simulink model "ElectricalSystems"  (R2020a)
settings: Solver=ode23t  StartTime=0.0  StopTime=10  RelTol=1e-3
undefined symbols (not defined in the file or in its folder): a, J, Ke, kt, kv, R, sigbuilder_block, Ts_motor, w0
libraries: fl_lib x54, nesl_utility x44, ee_lib x20, powerlib_meascontrol x16, fl_ps_legacy_lib x4, simulink x3
(part 2 of 2)

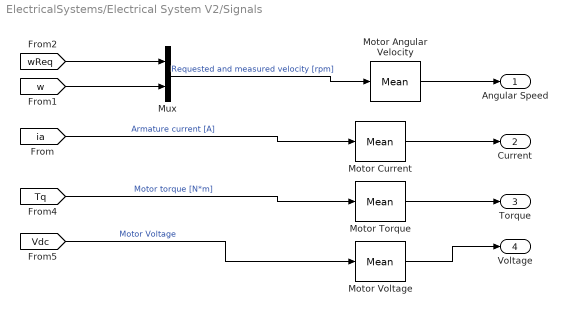
== system ElectricalSystems/Electrical System V2/Signals ==
  Motor Angular Velocity : powerlib_meascontrol/Measurements/Mean  Freq=100  Vinit=0  Ts=0
  Motor Current : powerlib_meascontrol/Measurements/Mean  Freq=100  Vinit=0  Ts=0
  Motor Torque : powerlib_meascontrol/Measurements/Mean  Freq=100  Vinit=0  Ts=0
  Motor Voltage : powerlib_meascontrol/Measurements/Mean  Freq=100  Vinit=0  Ts=0
  Mux : Mux  Inputs=2
  Angular Speed : Outport  VectorParamsAs1DForOutWhenUnconnected=off
  Current : Outport  Port=2  VectorParamsAs1DForOutWhenUnconnected=off
  Torque : Outport  Port=3  VectorParamsAs1DForOutWhenUnconnected=off
  Voltage : Outport  Port=4  VectorParamsAs1DForOutWhenUnconnected=off
  wires:
  [Tq] -> Motor Torque/1  "Motor torque [N*m]"
  [w] -> Mux/2
  Mux/1 -> Motor Angular Velocity/1  "Requested and measured velocity [rpm]"
  [wReq] -> Mux/1
  [ia] -> Motor Current/1  "Armature current [A]"
  [Vdc] -> Motor Voltage/1  "Motor Voltage"
  Motor Angular Velocity/1 -> Angular Speed/1
  Motor Current/1 -> Current/1
  Motor Torque/1 -> Torque/1
  Motor Voltage/1 -> Voltage/1

== system ElectricalSystems/Electrical System V3/Aero Drag ==
  Aerodynamic Drag : fl_lib/Mechanical/Mechanical Sources/Ideal Torque Source
      settings: SourceProductBaseCode=MT,SS
  Ideal Torque Sensor1 : fl_lib/Mechanical/Mechanical Sensors/Ideal Torque Sensor
  Motion Sensor : fl_lib/Mechanical/Mechanical Sensors/Ideal Rotational Motion Sensor  wrap_angle=simscape.enum.onoff.off  offset=0 deg
      settings: SourceProductBaseCode=MT,SS
  PS Terminator : fl_lib/Physical Signals/Sinks/PS Terminator
      settings: SourceProductBaseCode=MT,SS
  PS-Simulink Converter : nesl_utility/PS-Simulink Converter  PhysicalDomain=network_engine_domain  SubClassName=ps_output  LeftPortType=input  RightPortType=output  PseudoPeriodic=off  Frequencies=[]  Unit=inherit  AffineConversion=off
  RPM to Resistive Torque and Thrust : Subsystem
  Simulink-PS Converter : nesl_utility/Simulink-PS Converter  PhysicalDomain=network_engine_domain  SubClassName=ps_input  LeftPortType=input  RightPortType=output  PseudoPeriodic=off  Frequencies=[]  NoiseDistribution=none  NoiseParameters=[]  Unit=1  AffineConversion=off  FilteringAndDerivatives=provide  SimscapeFilterOrder=1  InputFilterTimeConstant=0.001  UdotUserProvided=0
  Terminator : Terminator
  R : PMIOPort  Side=Left
  C : PMIOPort  Port=2  Side=Right
  tag scope: Thrust1=global, Torque1=global
  wires:
  PS-Simulink Converter/1 -> Terminator/1  "Resistive Torque"
  RPM to Resistive Torque and Thrust/1(Thrust) -> [Thrust1]  "Thrust"
  RPM to Resistive Torque and Thrust/2(Resistive Torque) -> Simulink-PS Converter/1, [Torque1]
  connections:
  PS Terminator/LConn1 -- Motion Sensor/RConn3
  Motion Sensor/RConn1 -- C/RConn1 -- Aerodynamic Drag/RConn2
  Motion Sensor/LConn1 -- Ideal Torque Sensor1/LConn1 -- Aerodynamic Drag/LConn1
  Ideal Torque Sensor1/RConn1 -- R/RConn1
  PS-Simulink Converter/LConn1 -- Ideal Torque Sensor1/RConn2
  RPM to Resistive Torque and Thrust/LConn1 -- Motion Sensor/RConn2
  Simulink-PS Converter/RConn1 -- Aerodynamic Drag/RConn1

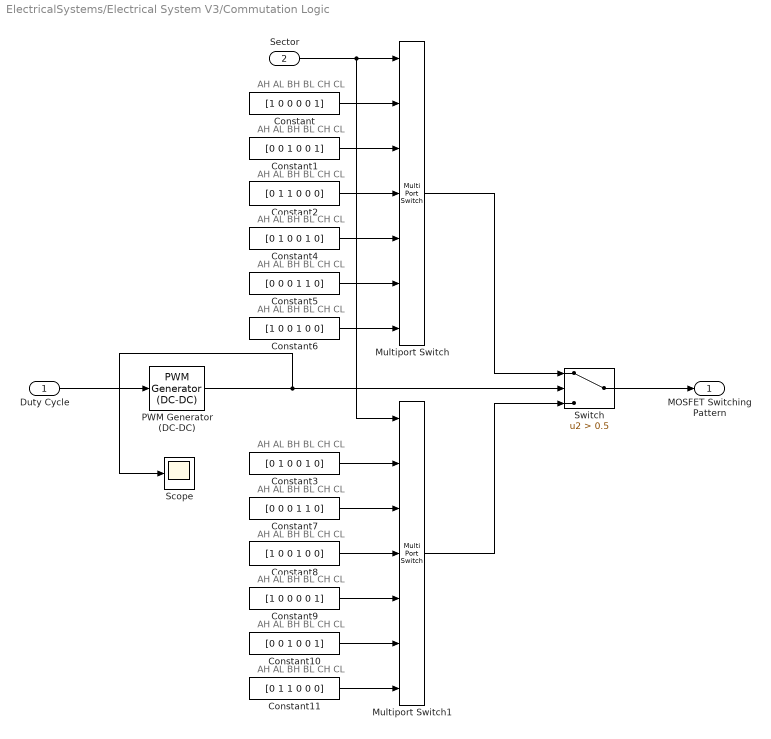
== system ElectricalSystems/Electrical System V3/Commutation Logic ==
  note: AH AL BH BL CH CL
  note: AH AL BH BL CH CL
  note: AH AL BH BL CH CL
  note: AH AL BH BL CH CL
  note: AH AL BH BL CH CL
  note: AH AL BH BL CH CL
  note: AH AL BH BL CH CL
  note: AH AL BH BL CH CL
  note: AH AL BH BL CH CL
  note: AH AL BH BL CH CL
  note: AH AL BH BL CH CL
  note: AH AL BH BL CH CL
  Duty Cycle : Inport
  Sector : Inport  Port=2
  Constant : Constant  Value=[1 0 0 0 0 1]
  Constant1 : Constant  Value=[0 0 1 0 0 1]
  Constant10 : Constant  Value=[0 0 1 0 0 1]
  Constant11 : Constant  Value=[0 1 1 0 0 0]
  Constant2 : Constant  Value=[0 1 1 0 0 0]
  Constant3 : Constant  Value=[0 1 0 0 1 0]
  Constant4 : Constant  Value=[0 1 0 0 1 0]
  Constant5 : Constant  Value=[0 0 0 1 1 0]
  Constant6 : Constant  Value=[1 0 0 1 0 0]
  Constant7 : Constant  Value=[0 0 0 1 1 0]
  Constant8 : Constant  Value=[1 0 0 1 0 0]
  Constant9 : Constant  Value=[1 0 0 0 0 1]
  Multiport Switch : MultiPortSwitch  Inputs=6
  Multiport Switch1 : MultiPortSwitch  Inputs=6
  PWM Generator (DC-DC) : powerlib_meascontrol/Pulse & Signal Generators/PWM Generator (DC-DC)  Fsw=50  Ts=Ts_motor
  Scope : Scope
  Switch : Switch  Criteria=u2 > Threshold  Threshold=0.5
  "  MOSFET Switching Pattern" : Outport  VectorParamsAs1DForOutWhenUnconnected=off
  wires:
  Sector/1 -> Multiport Switch1/1, Multiport Switch/1
  Constant10/1 -> Multiport Switch1/6
  Constant3/1 -> Multiport Switch1/2
  Constant6/1 -> Multiport Switch/7
  Constant/1 -> Multiport Switch/2
  Constant4/1 -> Multiport Switch/5
  Constant7/1 -> Multiport Switch1/3
  Constant5/1 -> Multiport Switch/6
  Constant2/1 -> Multiport Switch/4
  Constant1/1 -> Multiport Switch/3
  PWM Generator (DC-DC)/1 -> Scope/1, Switch/2
  Constant8/1 -> Multiport Switch1/4
  Multiport Switch1/1 -> Switch/3
  Multiport Switch/1 -> Switch/1
  Duty Cycle/1 -> PWM Generator (DC-DC)/1
  Switch/1 -> "  MOSFET Switching Pattern"/1
  Constant9/1 -> Multiport Switch1/5
  Constant11/1 -> Multiport Switch1/7

== system ElectricalSystems/Electrical System V3/Controller ==
  Error : Inport
  Discrete PID Controller : simulink/Continuous/PID Controller  Controller=P  Form=Parallel  TimeDomain=Continuous-time  UseExternalTs=off  SampleTime=Ts_motor  IntegratorMethod=Forward Euler  FilterMethod=Forward Euler  ControllerParametersSource=internal  P=1  I=0.1  D=0  UseFilter=on  N=100  TunerSelectOption=Transfer Function Based (PID Tuner App)  InitialConditionSource=internal  InitialConditionForIntegrator=0  InitialConditionForFilter=0  DifferentiatorICPrevScaledInput=0  ExternalReset=none  TrackingMode=off  Kt=1  LimitOutput=off  UpperSaturationLimit=1  LowerSaturationLimit=0.5  LinearizeAsGain=off  AntiWindupMode=back-calculation  Kb=1  POutMin=[]  POutMax=[]  IOutMin=[]  IOutMax=[]  DOutMin=[]  DOutMax=[]  NOutMin=[]  NOutMax=[]  SumOutMin=[]  SumOutMax=[]  SaturationOutMin=[]  SaturationOutMax=[]  PParamMin=[]  PParamMax=[]  IParamMin=[]  IParamMax=[]  DParamMin=[]  DParamMax=[]  NParamMin=[]  NParamMax=[]  KbParamMin=[]  KbParamMax=[]  KtParamMin=[]  KtParamMax=[]  KbOutMin=[]  KbOutMax=[]  KtOutMin=[]  KtOutMax=[]  IntegratorOutMin=[]  IntegratorOutMax=[]  FilterOutMin=[]  FilterOutMax=[]  SumI1OutMin=[]  SumI1OutMax=[]  SumI2OutMin=[]  SumI2OutMax=[]  SumI3OutMin=[]  SumI3OutMax=[]  SumI4OutMin=[]  SumI4OutMax=[]  SumDOutMin=[]  SumDOutMax=[]  DifferentiatorOutMin=[]  DifferentiatorOutMax=[]  FilterDiffOutCoefMin=[]  FilterDiffOutCoefMax=[]  ReciprocalOutMin=[]  ReciprocalOutMax=[]  SumDenOutMin=[]  SumDenOutMax=[]  SumNumOutMin=[]  SumNumOutMax=[]  DivideOutMin=[]  DivideOutMax=[]  UdiffTsProdOutMin=[]  UdiffTsProdOutMax=[]  NTsProdOutMin=[]  NTsProdOutMax=[]  UintegralTsProdOutMin=[]  UintegralTsProdOutMax=[]  UngainTsProdOutMin=[]  UngainTsProdOutMax=[]  IntegratorContinuousStateAttributes=''  IntegratorStateMustResolveToSignalObject=off  IntegratorRTWStateStorageClass=Auto  FilterContinuousStateAttributes=''  FilterStateMustResolveToSignalObject=off  FilterRTWStateStorageClass=Auto  ParallelPVariant=InternalParameters  IdealPVariant=Disabled  IVariant=Disabled  DVariant=Disabled  IntegratorVariant=Disabled  SatVariant=Disabled  AWVariant=Disabled  PCopyVariant=Disabled  TRVariant=Disabled  FdbkBlocksVariant=Forward  IdealPFdbkVariant=Disabled  SatFdbkVariant=Disabled  DerivativeFilterVariant=Disabled  NVariant=Disabled  NCopyVariant=Disabled_SignalSpec  FilterICVariant=Disabled  IntegratorICVariant=Disabled  ExternalResetVariant=Disabled  TRSumVariant=Passthrough  SumFdbkVariant=Disabled  SumVariant=Passthrough_P  TsampFilterVariant=InternalTs  TsampNgainVariant=Passthrough  TsampIntegralVariant=Disabled_SignalSpec
  Duty Cycle : Outport
  wires:
  Discrete PID Controller/1 -> Duty Cycle/1
  Error/1 -> Discrete PID Controller/1

== system ElectricalSystems/Electrical System V3/Desired speed ==
  Repeating Sequence Interpolated1 : simulink/Sources/Repeating Sequence Interpolated  OutValues=[0 4000 7000 7000 7000 7000]  TimeValues=[0 1 2 3 4 5]  LookUpMeth=Interpolation-Use End Values  tsamp=Ts_motor  OutMin=[]  OutMax=[]  OutDataTypeStr=double  OutputDataTypeScalingMode=double  OutDataType=fixdt(0,8)  OutScaling=2^-10
  Out1 : Outport
  Desired Speed : Outport  Port=2
  wires:
  Repeating Sequence Interpolated1/1 -> Desired Speed/1, Out1/1

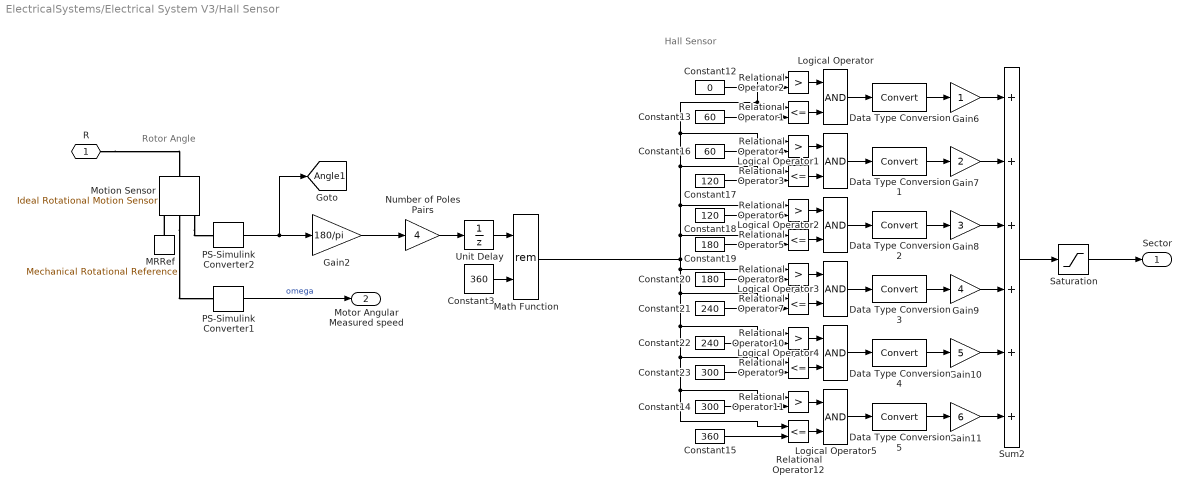
== system ElectricalSystems/Electrical System V3/Hall Sensor ==
  note: Rotor Angle
  note: Hall Sensor
  Constant12 : Constant  Value=0
  Constant13 : Constant  Value=60
  Constant14 : Constant  Value=300
  Constant15 : Constant  Value=360
  Constant16 : Constant  Value=60
  Constant17 : Constant  Value=120
  Constant18 : Constant  Value=120
  Constant19 : Constant  Value=180
  Constant20 : Constant  Value=180
  Constant21 : Constant  Value=240
  Constant22 : Constant  Value=240
  Constant23 : Constant  Value=300
  Constant3 : Constant  Value=360
  Data Type Conversion{,1..5} (6 alike) : DataTypeConversion  SaturateOnIntegerOverflow=on  RndMeth=Zero
  Gain10 : Gain  Gain=5  SaturateOnIntegerOverflow=on  OutDataTypeStr=Inherit: Same as input  ParamDataTypeStr=Inherit: Same as input
  Gain11 : Gain  Gain=6  SaturateOnIntegerOverflow=on  OutDataTypeStr=Inherit: Same as input  ParamDataTypeStr=Inherit: Same as input
  Gain2 : Gain  Gain=180/pi
  Gain6 : Gain  SaturateOnIntegerOverflow=on  OutDataTypeStr=Inherit: Same as input  ParamDataTypeStr=Inherit: Same as input
  Gain7 : Gain  Gain=2  SaturateOnIntegerOverflow=on  OutDataTypeStr=Inherit: Same as input  ParamDataTypeStr=Inherit: Same as input
  Gain8 : Gain  Gain=3  SaturateOnIntegerOverflow=on  OutDataTypeStr=Inherit: Same as input  ParamDataTypeStr=Inherit: Same as input
  Gain9 : Gain  Gain=4  SaturateOnIntegerOverflow=on  OutDataTypeStr=Inherit: Same as input  ParamDataTypeStr=Inherit: Same as input
  Logical Operator{,1..5} (6 alike) : Logic
  MRRef : fl_lib/Mechanical/Rotational Elements/Mechanical Rotational Reference
      settings: SourceProductName=Foundation Library
  Math Function : Math  Operator=rem  SignedPower=on  SaturateOnIntegerOverflow=on
  Motion Sensor : fl_lib/Mechanical/Mechanical Sensors/Ideal Rotational Motion Sensor  wrap_angle=simscape.enum.onoff.off  offset=0 deg
      settings: SourceProductName=Foundation Library
  Number of Poles Pairs : Gain  Gain=4
  PS-Simulink Converter1 : nesl_utility/PS-Simulink Converter  PhysicalDomain=network_engine_domain  SubClassName=ps_output  LeftPortType=input  RightPortType=output  PseudoPeriodic=off  Frequencies=[]  Unit=rpm  AffineConversion=off
      settings: SourceProductBaseCode=MT,SS
  PS-Simulink Converter2 : nesl_utility/PS-Simulink Converter  PhysicalDomain=network_engine_domain  SubClassName=ps_output  LeftPortType=input  RightPortType=output  PseudoPeriodic=off  Frequencies=[]  Unit=rad  AffineConversion=off
      settings: SourceProductBaseCode=MT,SS
  Relational Operator{1,3,5,7,9,12} (6 alike) : RelationalOperator  Operator=<=  RndMeth=Nearest  InputSameDT=on
  Relational Operator{2,4,6,8,10..11} (6 alike) : RelationalOperator  Operator=>  RndMeth=Nearest  InputSameDT=on
  Saturation : Saturate  UpperLimit=6  LowerLimit=1
  Sum2 : Sum  Inputs=++++++  InputSameDT=on  SaturateOnIntegerOverflow=on  OutDataTypeStr=Inherit: Same as first input
  Unit Delay : UnitDelay  SampleTime=Ts_motor  HasFrameUpgradeWarning=on
  R : PMIOPort  Side=Left
  Sector : Outport
  Motor Angular Measured speed : Outport  Port=2
  tag scope: Angle1=global
  wires:
  Math Function/1 -> Relational Operator2/1, Relational Operator1/1, Relational Operator4/1, Relational Operator3/1, Relational Operator6/1, Relational Operator5/1, Relational Operator12/1, Relational Operator11/1, Relational Operator9/1, Relational Operator10/1, Relational Operator7/1, Relational Operator8/1
  Logical Operator1/1 -> Data Type Conversion1/1
  Logical Operator4/1 -> Data Type Conversion4/1
  Constant21/1 -> Relational Operator7/2
  Logical Operator5/1 -> Data Type Conversion5/1
  Constant15/1 -> Relational Operator12/2
  Constant3/1 -> Math Function/2
  Sum2/1 -> Saturation/1
  Logical Operator3/1 -> Data Type Conversion3/1
  Gain8/1 -> Sum2/3
  Constant12/1 -> Relational Operator2/2
  Gain2/1 -> Number of Poles Pairs/1
  Relational Operator12/1 -> Logical Operator5/2
  Gain9/1 -> Sum2/4
  Data Type Conversion4/1 -> Gain10/1
  Relational Operator7/1 -> Logical Operator3/2
  Gain10/1 -> Sum2/5
  Constant23/1 -> Relational Operator9/2
  Data Type Conversion/1 -> Gain6/1
  Relational Operator6/1 -> Logical Operator2/1
  Data Type Conversion3/1 -> Gain9/1
  Data Type Conversion1/1 -> Gain7/1
  Constant18/1 -> Relational Operator6/2
  Relational Operator9/1 -> Logical Operator4/2
  Unit Delay/1 -> Math Function/1
  Constant19/1 -> Relational Operator5/2
  Logical Operator/1 -> Data Type Conversion/1
  Relational Operator10/1 -> Logical Operator4/1
  Saturation/1 -> Sector/1
  Constant13/1 -> Relational Operator1/2
  Gain6/1 -> Sum2/1
  Relational Operator4/1 -> Logical Operator1/1
  Relational Operator2/1 -> Logical Operator/1
  Constant22/1 -> Relational Operator10/2
  Data Type Conversion5/1 -> Gain11/1
  Constant17/1 -> Relational Operator3/2
  Relational Operator5/1 -> Logical Operator2/2
  Relational Operator1/1 -> Logical Operator/2
  Relational Operator11/1 -> Logical Operator5/1
  Gain7/1 -> Sum2/2
  Relational Operator3/1 -> Logical Operator1/2
  Data Type Conversion2/1 -> Gain8/1
  Number of Poles Pairs/1 -> Unit Delay/1
  Constant14/1 -> Relational Operator11/2
  Constant20/1 -> Relational Operator8/2
  PS-Simulink Converter2/1 -> [Angle1], Gain2/1
  PS-Simulink Converter1/1 -> Motor Angular Measured speed/1  "omega"
  Logical Operator2/1 -> Data Type Conversion2/1
  Constant16/1 -> Relational Operator4/2
  Gain11/1 -> Sum2/6
  Relational Operator8/1 -> Logical Operator3/1
  connections:
  MRRef/LConn1 -- Motion Sensor/RConn1
  R/RConn1 -- Motion Sensor/LConn1
  Motion Sensor/RConn3 -- PS-Simulink Converter2/LConn1
  Motion Sensor/RConn2 -- PS-Simulink Converter1/LConn1

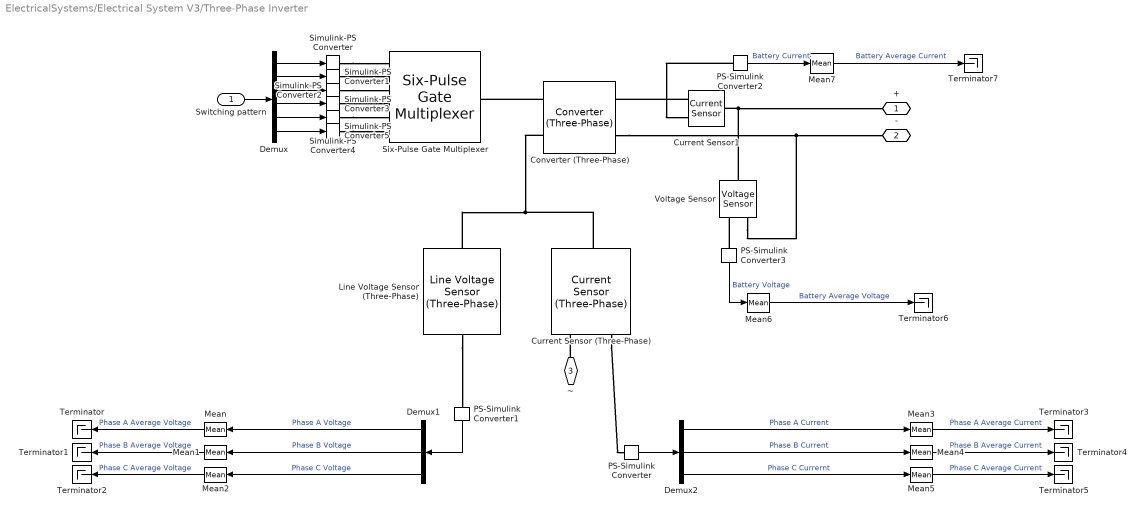
== system ElectricalSystems/Electrical System V3/Three-Phase Inverter ==
  Switching pattern : Inport
  Converter (Three-Phase) : ee_lib/Semiconductors & Converters/Converters/Converter (Three-Phase)  device_type=ee.enum.converters.switchingdevice.mosfet  Vf=0.8 V  Ron=0.000001 Ohm  Rds=0.001 Ohm  Goff=0.001 1/Ohm  Vth=0.3 V  Vgt=1 V  Vgt_off=-1 V  Ih=1 A  diode_param=ee.enum.converters.protectiondiode.none  diode_Vf=0.8 V  diode_Ron=0.001 Ohm  diode_Goff=1e-5 1/Ohm  diode_C=50 nF  diode_iRM=-235 A  diode_iF=300 A  diode_idot=-50 A/us  diode_trr_param=ee.enum.converters.diodetrr.trr_factor  diode_trr_factor=3  diode_trr=15 us  diode_Qrr=1500 s*uA  snubber_type=ee.enum.converters.snubber.exclude  Rs=0.1 Ohm  Cs=1e-7 F
      settings: SourceProductBaseCode=PS
  Current Sensor (Three-Phase) : ee_lib/Sensors & Transducers/Current Sensor (Three-Phase)
  Current Sensor1 : fl_lib/Electrical/Electrical Sensors/Current Sensor
  Demux : Demux  Outputs=6
  Demux1 : Demux  Outputs=3
  Demux2 : Demux  Outputs=3
  Line Voltage Sensor (Three-Phase) : ee_lib/Sensors & Transducers/Line Voltage Sensor (Three-Phase)
      settings: SourceProductBaseCode=PS
  Mean{,1..7} (8 alike) : powerlib_meascontrol/Measurements/Mean  Freq=50  Vinit=0  Ts=Ts_motor
  PS-Simulink Converter : nesl_utility/PS-Simulink Converter  PhysicalDomain=network_engine_domain  SubClassName=ps_output  LeftPortType=input  RightPortType=output  PseudoPeriodic=off  Frequencies=[]  Unit=1  AffineConversion=off
      settings: SourceProductBaseCode=MT,SS
  PS-Simulink Converter1 : nesl_utility/PS-Simulink Converter  PhysicalDomain=network_engine_domain  SubClassName=ps_output  LeftPortType=input  RightPortType=output  PseudoPeriodic=off  Frequencies=[]  Unit=1  AffineConversion=off
      settings: SourceProductBaseCode=MT,SS
  PS-Simulink Converter2 : nesl_utility/PS-Simulink Converter  PhysicalDomain=network_engine_domain  SubClassName=ps_output  LeftPortType=input  RightPortType=output  PseudoPeriodic=off  Frequencies=[]  Unit=inherit  AffineConversion=off
  PS-Simulink Converter3 : nesl_utility/PS-Simulink Converter  PhysicalDomain=network_engine_domain  SubClassName=ps_output  LeftPortType=input  RightPortType=output  PseudoPeriodic=off  Frequencies=[]  Unit=inherit  AffineConversion=off
  Simulink-PS Converter{,1..5} (6 alike) : nesl_utility/Simulink-PS Converter  PhysicalDomain=network_engine_domain  SubClassName=ps_input  LeftPortType=input  RightPortType=output  PseudoPeriodic=off  Frequencies=[]  NoiseDistribution=none  NoiseParameters=[]  Unit=1  AffineConversion=off  FilteringAndDerivatives=provide  SimscapeFilterOrder=1  InputFilterTimeConstant=0.001  UdotUserProvided=0
      settings: SourceProductBaseCode=MT,SS
  Six-Pulse Gate Multiplexer : ee_lib/Semiconductors & Converters/Converters/Six-Pulse Gate Multiplexer  R=0 Ohm
      settings: SourceProductBaseCode=PS  InternalSimscapePortConfiguration="{\"Bottom\":[],\"Left\":[{\"id\":\"GaH\",\"label\":\"Ga(H)\",\"type\":\"input\"},{\"id\":\"GaL\",\"label\":\"Ga(L)\",\"type\":\"input\"},{\"id\":\"GbH\",\"label\":\"Gb(H)\",\"type\":\"input\"},{\"id\":\"GbL\",\"label\":\"Gb(L)\",\"type\":\"input\"},{\"id\":\"GcH\",\"label\":\"Gc(H)\",\"type\":\"input\"},{\"id\":\"GcL\",\"label\":\"Gc(L)\",\"type\":\"input\"}],\"Right\":[{\"id\":\"p\",\"label\":\"G\",\"type\":\"foundation.electrical.twelve_phase\"}],\"Top\":[]}"
  Terminator{,1..7} (8 alike) : Terminator
  Voltage Sensor : fl_lib/Electrical/Electrical Sensors/Voltage Sensor
  + : PMIOPort  Side=Left
  - : PMIOPort  Port=2  Side=Left
  ~ : PMIOPort  Port=3  Side=Right
  wires:
  Switching pattern/1 -> Demux/1
  Demux/1 -> Simulink-PS Converter/1
  Demux/2 -> Simulink-PS Converter1/1
  Demux/3 -> Simulink-PS Converter2/1
  Demux/4 -> Simulink-PS Converter3/1
  Demux/5 -> Simulink-PS Converter4/1
  Demux/6 -> Simulink-PS Converter5/1
  PS-Simulink Converter2/1 -> Mean7/1  "Battery Current"
  PS-Simulink Converter3/1 -> Mean6/1  "Battery Voltage"
  Demux1/1 -> Mean/1  "Phase A Voltage"
  Demux1/3 -> Mean2/1  "Phase C Voltage"
  PS-Simulink Converter1/1 -> Demux1/1
  Demux1/2 -> Mean1/1  "Phase B Voltage"
  PS-Simulink Converter/1 -> Demux2/1
  Demux2/1 -> Mean3/1  "Phase A Current"
  Demux2/2 -> Mean4/1  "Phase B Current"
  Demux2/3 -> Mean5/1  "Phase C Currernt"
  Mean/1 -> Terminator/1  "Phase A Average Voltage"
  Mean1/1 -> Terminator1/1  "Phase B Average Voltage"
  Mean2/1 -> Terminator2/1  "Phase C Average Voltage"
  Mean3/1 -> Terminator3/1  "Phase A Average Current"
  Mean4/1 -> Terminator4/1  "Phase B Average Current"
  Mean5/1 -> Terminator5/1  "Phase C Average Current"
  Mean6/1 -> Terminator6/1  "Battery Average Voltage"
  Mean7/1 -> Terminator7/1  "Battery Average Current"
  connections:
  Current Sensor (Three-Phase)/RConn1 -- PS-Simulink Converter/LConn1
  Simulink-PS Converter/RConn1 -- Six-Pulse Gate Multiplexer/LConn1
  Simulink-PS Converter1/RConn1 -- Six-Pulse Gate Multiplexer/LConn2
  Simulink-PS Converter2/RConn1 -- Six-Pulse Gate Multiplexer/LConn3
  Simulink-PS Converter3/RConn1 -- Six-Pulse Gate Multiplexer/LConn4
  Simulink-PS Converter4/RConn1 -- Six-Pulse Gate Multiplexer/LConn5
  Simulink-PS Converter5/RConn1 -- Six-Pulse Gate Multiplexer/LConn6
  Converter (Three-Phase)/LConn1 -- Six-Pulse Gate Multiplexer/RConn1
  Converter (Three-Phase)/RConn2 -- Voltage Sensor/RConn2 -- -/RConn1
  Line Voltage Sensor (Three-Phase)/LConn1 -- Converter (Three-Phase)/LConn2 -- Current Sensor (Three-Phase)/LConn1
  Line Voltage Sensor (Three-Phase)/RConn1 -- PS-Simulink Converter1/LConn1
  ~/RConn1 -- Current Sensor (Three-Phase)/RConn2
  Current Sensor1/RConn2 -- Converter (Three-Phase)/RConn1
  Voltage Sensor/LConn1 -- +/RConn1 -- Current Sensor1/LConn1
  PS-Simulink Converter2/LConn1 -- Current Sensor1/RConn1
  PS-Simulink Converter3/LConn1 -- Voltage Sensor/RConn1

== system ElectricalSystems/Electrical System V4/RPM to Resistive Torque and Thrust ==
  Angular Speed : Inport
  Constant : Constant  Value=0
  From : From  Commented=on  GotoTag=Velocity  TagVisibility=global
  Gain : Gain  Gain=-1
  Saturation : Saturate  UpperLimit=15000  LowerLimit=0
  Thrust & Torque Based on Propeller Rotational and Translational Velocity : MATLAB Function  TreatAsAtomicUnit=on
  Thrust : Outport
  Resistive Torque : Outport  Port=2
  wires:
  Thrust & Torque Based on Propeller Rotational and Translational Velocity/1(Thrust) -> Thrust/1
  Angular Speed/1 -> Saturation/1  "Speed"
  Thrust & Torque Based on Propeller Rotational and Translational Velocity/2(Torque) -> Gain/1
  Constant/1 -> Thrust & Torque Based on Propeller Rotational and Translational Velocity/1(Velocity)
  Saturation/1 -> Thrust & Torque Based on Propeller Rotational and Translational Velocity/2(RPM)
  Gain/1 -> Resistive Torque/1

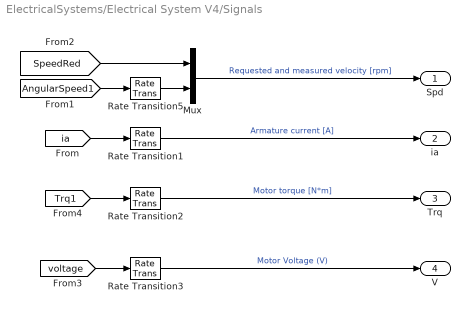
== system ElectricalSystems/Electrical System V4/Signals ==
  Mux : Mux  Inputs=2
  Rate Transition{1..3,5} (4 alike) : RateTransition
  Spd : Outport  VectorParamsAs1DForOutWhenUnconnected=off
  ia : Outport  Port=2  VectorParamsAs1DForOutWhenUnconnected=off
  Trq : Outport  Port=3  VectorParamsAs1DForOutWhenUnconnected=off
  V : Outport  Port=4  VectorParamsAs1DForOutWhenUnconnected=off
  wires:
  Rate Transition2/1 -> Trq/1  "Motor torque [N*m]"
  [ia] -> Rate Transition1/1
  [AngularSpeed1] -> Rate Transition5/1
  [Trq1] -> Rate Transition2/1
  Rate Transition5/1 -> Mux/2
  Mux/1 -> Spd/1  "Requested and measured velocity [rpm]"
  [SpeedRed] -> Mux/1
  Rate Transition1/1 -> ia/1  "Armature current [A]"
  [voltage] -> Rate Transition3/1
  Rate Transition3/1 -> V/1  "Motor Voltage (V)"

== system ElectricalSystems/Electrical System V5/RPM to Resistive Torque and Thrust ==
  Angular Speed : Inport
  Constant : Constant  Value=0
  From : From  Commented=on  GotoTag=Velocity  TagVisibility=global
  Gain : Gain  Gain=-1
  Saturation : Saturate  UpperLimit=15000  LowerLimit=0
  Thrust & Torque Based on Propeller Rotational and Translational Velocity : MATLAB Function  TreatAsAtomicUnit=on
  Thrust : Outport
  Resistive Torque : Outport  Port=2
  wires:
  Gain/1 -> Resistive Torque/1
  Saturation/1 -> Thrust & Torque Based on Propeller Rotational and Translational Velocity/2(RPM)
  Constant/1 -> Thrust & Torque Based on Propeller Rotational and Translational Velocity/1(Velocity)
  Thrust & Torque Based on Propeller Rotational and Translational Velocity/2(Torque) -> Gain/1
  Angular Speed/1 -> Saturation/1  "Speed"
  Thrust & Torque Based on Propeller Rotational and Translational Velocity/1(Thrust) -> Thrust/1

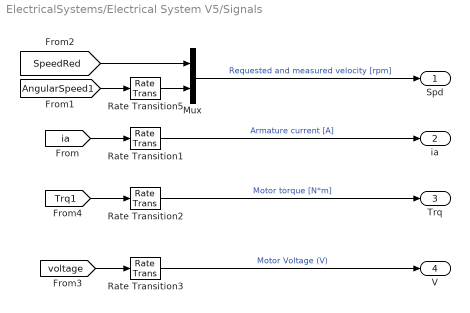
== system ElectricalSystems/Electrical System V5/Signals ==
  Mux : Mux  Inputs=2
  Rate Transition{1..3,5} (4 alike) : RateTransition
  Spd : Outport  VectorParamsAs1DForOutWhenUnconnected=off
  ia : Outport  Port=2  VectorParamsAs1DForOutWhenUnconnected=off
  Trq : Outport  Port=3  VectorParamsAs1DForOutWhenUnconnected=off
  V : Outport  Port=4  VectorParamsAs1DForOutWhenUnconnected=off
  wires:
  Rate Transition3/1 -> V/1  "Motor Voltage (V)"
  [voltage] -> Rate Transition3/1
  Rate Transition1/1 -> ia/1  "Armature current [A]"
  [SpeedRed] -> Mux/1
  Mux/1 -> Spd/1  "Requested and measured velocity [rpm]"
  Rate Transition5/1 -> Mux/2
  [Trq1] -> Rate Transition2/1
  [AngularSpeed1] -> Rate Transition5/1
  [ia] -> Rate Transition1/1
  Rate Transition2/1 -> Trq/1  "Motor torque [N*m]"

== system ElectricalSystems/Electrical System V1/Aero Drag/Square law ==
  Nm/(rad/s)^2 : fl_ps_legacy_lib/Legacy Physical Signals/Functions/PS Gain  gain=-8e-8
      settings: SourceProductBaseCode=MT,SS
  PS Product : fl_ps_legacy_lib/Legacy Physical Signals/Functions/PS Product
      settings: SourceProductBaseCode=MT,SS
  w : PMIOPort  Side=Left
  trq : PMIOPort  Port=2  Side=Right
  connections:
  w/RConn1 -- PS Product/LConn2 -- PS Product/LConn1
  Nm/(rad/s)^2/RConn1 -- trq/RConn1
  PS Product/RConn1 -- Nm/(rad/s)^2/LConn1

== system ElectricalSystems/Electrical System V2/Aero Drag/Square law ==
  Nm/(rad/s)^2 : fl_ps_legacy_lib/Legacy Physical Signals/Functions/PS Gain  gain=-8e-8
      settings: SourceProductBaseCode=MT,SS
  PS Product : fl_ps_legacy_lib/Legacy Physical Signals/Functions/PS Product
      settings: SourceProductBaseCode=MT,SS
  w : PMIOPort  Side=Left
  trq : PMIOPort  Port=2  Side=Right
  connections:
  w/RConn1 -- PS Product/LConn2 -- PS Product/LConn1
  Nm/(rad/s)^2/RConn1 -- trq/RConn1
  PS Product/RConn1 -- Nm/(rad/s)^2/LConn1

== system ElectricalSystems/Electrical System V3/Aero Drag/RPM to Resistive Torque and Thrust ==
  Constant : Constant  Value=0
  From : From  Commented=on  GotoTag=Velocity  TagVisibility=global
  PS-Simulink Converter1 : nesl_utility/PS-Simulink Converter  PhysicalDomain=network_engine_domain  SubClassName=ps_output  LeftPortType=input  RightPortType=output  PseudoPeriodic=off  Frequencies=[]  Unit=rpm  AffineConversion=off
  Thrust & Torque Based on Propeller Rotational and Translational Velocity : MATLAB Function  TreatAsAtomicUnit=on
  Unit Delay : UnitDelay  SampleTime=-1  HasFrameUpgradeWarning=on
  Angular Speed : PMIOPort  Side=Left
  Thrust : Outport
  Resistive Torque : Outport  Port=2
  wires:
  Thrust & Torque Based on Propeller Rotational and Translational Velocity/1(Thrust) -> Thrust/1
  PS-Simulink Converter1/1 -> Unit Delay/1  "Speed2"
  Unit Delay/1 -> Thrust & Torque Based on Propeller Rotational and Translational Velocity/2(RPM)
  Thrust & Torque Based on Propeller Rotational and Translational Velocity/2(Torque) -> Resistive Torque/1
  Constant/1 -> Thrust & Torque Based on Propeller Rotational and Translational Velocity/1(Velocity)
  connections:
  PS-Simulink Converter1/LConn1 -- Angular Speed/RConn1

== matlab function ElectricalSystems/Electrical System V3/Aero Drag/RPM to Resistive Torque and Thrust/Thrust & Torque Based on Propeller Rotational and Translational Velocity ==
  data: Thrust output; Velocity input; RPM input; Torque output
function [Thrust,Torque]= fcn(Velocity, RPM)

%Thrust
s1 = 0.07615;
s2 = 0.007241;
s3 = -7.12e-05;
s4 = -0.00219;
s5 = -1.683e-05;
s6 = 1.619e-07;
Thrust = s1 + s2*Velocity + s3*RPM + s4*Velocity.^2 + s5*Velocity.*RPM + s6*RPM.^2;

%Torque
k1 = 0.0003302;
k2 = 0.000295;
k3 = -1.33e-07;
k4 = -7.089e-05;
k5 = 7.352e-08;
k6 = 2.21e-09;
Torque = k1 + k2*Velocity + k3*RPM + k4*Velocity.^2 + k5*Velocity.*RPM + k6*RPM.^2;

== matlab function ElectricalSystems/Electrical System V4/RPM to Resistive Torque and Thrust/Thrust & Torque Based on Propeller Rotational and Translational Velocity ==
  data: Thrust output; Velocity input; RPM input; Torque output
function [Thrust,Torque]= fcn(Velocity, RPM)

%Thrust
s1 = 0.07615;
s2 = 0.007241;
s3 = -7.12e-05;
s4 = -0.00219;
s5 = -1.683e-05;
s6 = 1.619e-07;
Thrust = s1 + s2*Velocity + s3*RPM + s4*Velocity.^2 + s5*Velocity.*RPM + s6*RPM.^2;

%Torque
k1 = 0.0003302;
k2 = 0.000295;
k3 = -1.33e-07;
k4 = -7.089e-05;
k5 = 7.352e-08;
k6 = 2.21e-09;
Torque = k1 + k2*Velocity + k3*RPM + k4*Velocity.^2 + k5*Velocity.*RPM + k6*RPM.^2;

== matlab function ElectricalSystems/Electrical System V5/RPM to Resistive Torque and Thrust/Thrust & Torque Based on Propeller Rotational and Translational Velocity ==
  data: Thrust output; Velocity input; RPM input; Torque output
function [Thrust,Torque]= fcn(Velocity, RPM)

%Thrust
s1 = 0.07615;
s2 = 0.007241;
s3 = -7.12e-05;
s4 = -0.00219;
s5 = -1.683e-05;
s6 = 1.619e-07;
Thrust = s1 + s2*Velocity + s3*RPM + s4*Velocity.^2 + s5*Velocity.*RPM + s6*RPM.^2;

%Torque
k1 = 0.0003302;
k2 = 0.000295;
k3 = -1.33e-07;
k4 = -7.089e-05;
k5 = 7.352e-08;
k6 = 2.21e-09;
Torque = k1 + k2*Velocity + k3*RPM + k4*Velocity.^2 + k5*Velocity.*RPM + k6*RPM.^2;
